simulink model "Signal_Merge"  (R2021a)
settings: Solver=VariableStepAuto  StartTime=0.0  StopTime=10.0  RelTol=1e-3
settings Model: Creator=hp  LastModifiedBy=hp

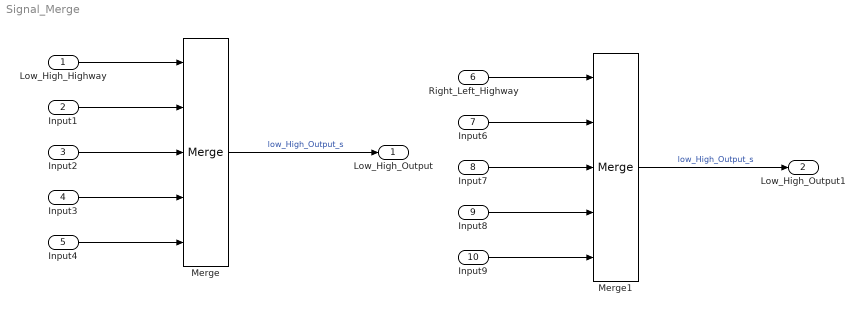
== system Signal_Merge ==
  Low_High_Highway : Inport
  Input1 : Inport  Port=2
  Input2 : Inport  Port=3
  Input3 : Inport  Port=4
  Input4 : Inport  Port=5
  Right_Left_Highway : Inport  Port=6
  Input6 : Inport  Port=7
  Input7 : Inport  Port=8
  Input8 : Inport  Port=9
  Input9 : Inport  Port=10
  Merge : Merge  Inputs=5
  Merge1 : Merge  Inputs=5
  Low_High_Output : Outport
  Low_High_Output1 : Outport  Port=2
  wires:
  Merge/1 -> Low_High_Output/1  "low_High_Output_s"
  Low_High_Highway/1 -> Merge/1
  Input1/1 -> Merge/2
  Input2/1 -> Merge/3
  Input3/1 -> Merge/4
  Input4/1 -> Merge/5
  Input9/1 -> Merge1/5
  Input7/1 -> Merge1/3
  Right_Left_Highway/1 -> Merge1/1
  Input6/1 -> Merge1/2
  Merge1/1 -> Low_High_Output1/1  "low_High_Output_s"
  Input8/1 -> Merge1/4
